simulink model "task1Model"  (Simulink 7.5)
settings: Solver=ode3  StartTime=0.0  StopTime=200  FixedStep=1  RelTol=1e-3
undefined symbols (not defined in the file): DiscIntNeverNeededParam, poissrnd
settings Model: Creator=Dranik_win  LastModifiedBy=Dranik_win

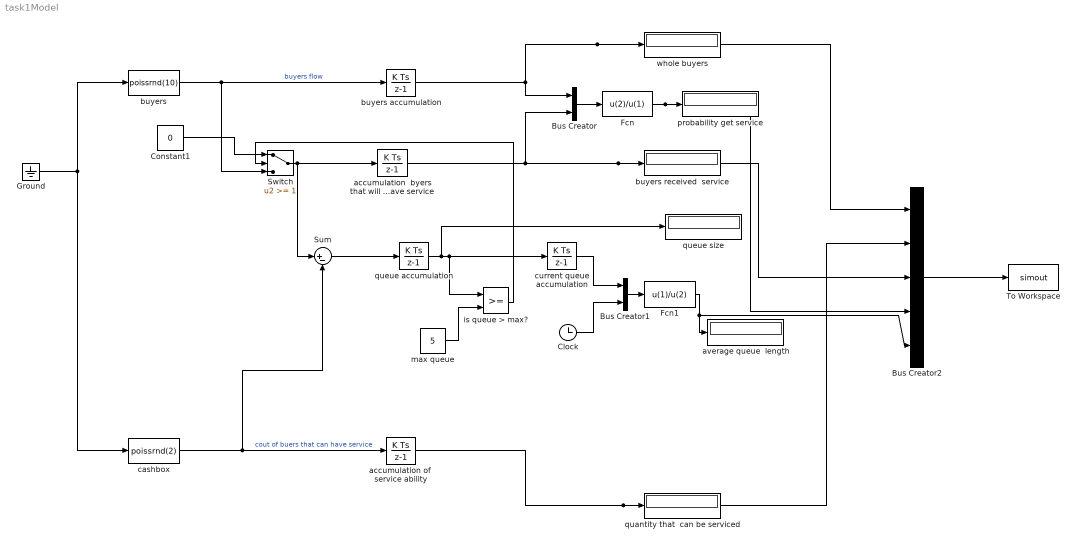
== system task1Model ==
  Bus Creator : BusCreator  Inputs=2
  Bus Creator1 : BusCreator  Inputs=2
  Bus Creator2 : BusCreator  Inputs=5
  Clock : Clock
      settings: Decimation=10
  Constant1 : Constant  Value=0  OutDataType=fixdt(1, 16)  OutScaling=2^0
  Fcn : Fcn  Expr=u(2)/u(1)
  Fcn1 : Fcn  Expr=u(1)/u(2)
  Ground : Ground
  Sum : Sum  Inputs=|+-  OutDataType=fixdt(1, 16)  OutScaling=2^0
  Switch : Switch  Threshold=1  OutDataType=fixdt(1, 16)  OutScaling=2^0
  To Workspace : ToWorkspace  VariableName=simout  SampleTime=-1  SaveFormat=Structure
  accumulation  byers that will have service : DiscreteIntegrator  OutDataType=fixdt(1, 16)  OutScaling=2^0  ICPrevOutput=DiscIntNeverNeededParam  ICPrevScaledInput=DiscIntNeverNeededParam
  "accumulation of  service ability " : DiscreteIntegrator  OutDataType=fixdt(1, 16)  OutScaling=2^0  ICPrevOutput=DiscIntNeverNeededParam  ICPrevScaledInput=DiscIntNeverNeededParam
  average queue  length : Display
  buyers : MATLABFcn  MATLABFcn=poissrnd(10)
  buyers accumulation : DiscreteIntegrator  OutDataType=fixdt(1, 16)  OutScaling=2^0  ICPrevOutput=DiscIntNeverNeededParam  ICPrevScaledInput=DiscIntNeverNeededParam
  buyers received  service : Display
  cashbox : MATLABFcn  MATLABFcn=poissrnd(2)
  current queue accumulation : DiscreteIntegrator  OutDataType=fixdt(1, 16)  OutScaling=2^0  ICPrevOutput=DiscIntNeverNeededParam  ICPrevScaledInput=DiscIntNeverNeededParam
  is queue > max? : RelationalOperator  LogicOutDataTypeMode=boolean  LogicDataType=fixdt(0, 8)  OutDataTypeStr=boolean
  max queue : Constant  Value=5  OutDataType=fixdt(1, 16)  OutScaling=2^0
  probability get service : Display
  quantity that  can be serviced : Display
  queue accumulation : DiscreteIntegrator  OutDataType=fixdt(1, 16)  OutScaling=2^0  LimitOutput=on  LowerSaturationLimit=0  ICPrevOutput=DiscIntNeverNeededParam  ICPrevScaledInput=DiscIntNeverNeededParam
  queue size : Display
  whole buyers : Display
  wires:
  Ground/1 -> buyers/1, cashbox/1
  buyers/1 -> buyers accumulation/1, Switch/3  "buyers flow"
  buyers accumulation/1 -> Bus Creator/1, whole buyers/1, Bus Creator2/1
  cashbox/1 -> "accumulation of  service ability "/1, Sum/2  "cout of buers that can have service"
  "accumulation of  service ability "/1 -> quantity that  can be serviced/1, Bus Creator2/2
  Sum/1 -> queue accumulation/1
  queue accumulation/1 -> queue size/1, is queue > max?/1, current queue accumulation/1
  max queue/1 -> is queue > max?/2
  is queue > max?/1 -> Switch/2
  Switch/1 -> Sum/1, accumulation  byers that will have service/1
  Constant1/1 -> Switch/1
  accumulation  byers that will have service/1 -> Bus Creator/2, buyers received  service/1, Bus Creator2/3
  Bus Creator/1 -> Fcn/1
  Fcn/1 -> probability get service/1, Bus Creator2/4
  current queue accumulation/1 -> Bus Creator1/1
  Clock/1 -> Bus Creator1/2
  Bus Creator1/1 -> Fcn1/1
  Fcn1/1 -> average queue  length/1, Bus Creator2/5
  Bus Creator2/1 -> To Workspace/1
